simulink model "P81s"  (R2015b)
settings: Solver=VariableStepAuto  StartTime=0.0  StopTime=1  RelTol=1e-3
settings Model: Creator=xmax1946  LastModifiedBy=xmax1946

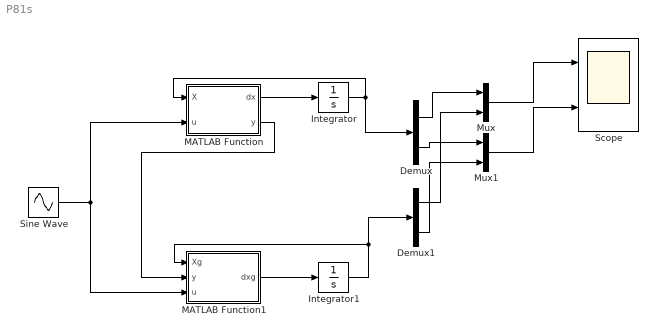
== system P81s ==
  Demux : Demux  Outputs=2
  Demux1 : Demux  Outputs=2
  Integrator : Integrator  InitialCondition=[100;10]
  Integrator1 : Integrator  InitialCondition=[pi;pi]
  MATLAB Function : MATLAB Function  TreatAsAtomicUnit=on
  MATLAB Function1 : MATLAB Function  TreatAsAtomicUnit=on
  Mux : Mux  Inputs=2
  Mux1 : Mux  Inputs=2
  Scope : Scope  NumInputPorts=2
  Sine Wave : Sin  Amplitude=10  SampleTime=0
  wires:
  MATLAB Function/1(dx) -> Integrator/1
  MATLAB Function1/1(dxg) -> Integrator1/1
  Integrator/1 -> MATLAB Function/1(X), Demux/1
  MATLAB Function/2(y) -> MATLAB Function1/2(y)
  Integrator1/1 -> Demux1/1, MATLAB Function1/1(Xg)
  Demux/1 -> Mux/1
  Demux1/1 -> Mux/2
  Demux/2 -> Mux1/1
  Demux1/2 -> Mux1/2
  Mux/1 -> Scope/1
  Mux1/1 -> Scope/2
  Sine Wave/1 -> MATLAB Function1/3(u), MATLAB Function/2(u)

== matlab function P81s/MATLAB Function1 ==
  data: Xg input; y input; u input; dxg output
function dxg =fcn(Xg,y,u)
A=[0,1;2,3];
B=[1;1];
C=[1,2];

L=[2;2];

dxg=A*Xg+B*u+L*(y-C*Xg);

== matlab function P81s/MATLAB Function ==
  data: dx output; X input; y output; u input
function [dx,y]=fcn(X,u)
A=[0,1;2,3];
B=[1;1];
C=[1,2];

dx=A*X+B*u;
y=C*X;
